simulink model "m13sol6"  (Simulink 7.7)
settings: Solver=ode45  StartTime=0.0  StopTime=10.0  RelTol=1e-3
undefined symbols (not defined in the file): seed61, seed62
settings Model: Creator=Esben  LastModifiedBy=Esben

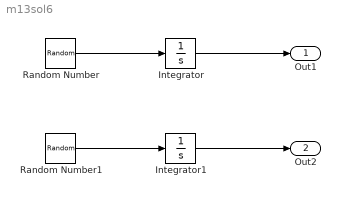
== system m13sol6 ==
  Integrator : Integrator
  Integrator1 : Integrator
  Random Number : RandomNumber  Seed=seed61  SampleTime=0.1
  Random Number1 : RandomNumber  Seed=seed62  SampleTime=0.1
  Out1 : Outport
  Out2 : Outport  Port=2
  wires:
  Random Number/1 -> Integrator/1
  Integrator/1 -> Out1/1
  Random Number1/1 -> Integrator1/1
  Integrator1/1 -> Out2/1
